simulink model "slexNLPClassificationLinearPredictExample"  (R2023a)
settings: Solver=FixedStepDiscrete  StartTime=0.0  StopTime=nlp.time(end)  FixedStep=1  RelTol=1e-3
PreLoadFcn:
  | if ~exist("linearMdl","var")
  | 
  | load nlpdata
  | 
  | n = size(X,1);
  | rng("default") % For reproducibility
  | shflidx = randperm(n);
  | X = X(shflidx,:);
  | Y = Y(shflidx);
  | 
  | Ystats = Y == "stats";
  | c = cvpartition(Ystats,Holdout=0.1);
  | idxPrsnt = training(c);
  | idxFtr = test(c);
  | 
  | prsntX = X(idxPrsnt,:);
  | prsntY = Ystats(idxPrsnt);
  | ftrX = X(idxFtr,:);
  | ftrY = Ystats(idxFtr);
  | 
  | linearMdl = fitclinear(prsntX,prsntY);
  | 
  | [nftrX,p] = size(ftrX);
  | nlp.time = (1:nftrX)' - 1;
  | nlp.signals(1).values = full(ftrX);
  | nlp.signals(1).dimensions = p;
  | 
  | end
libraries: statsLibrary x1
settings Model: Creator=The MathWorks, Inc.  LastModifiedBy=The MathWorks, Inc.
settings DataIOCC: ExternalInput=nlp  LoadExternalInput=on
settings OptimizationCC: ReuseModelBlockBuffer=off

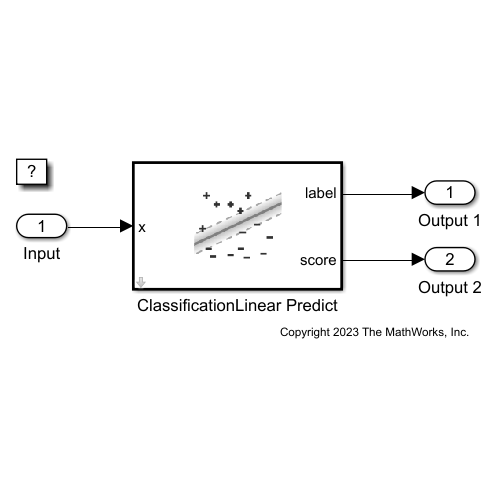
[thumbnail: Simulink's stored preview of the top-level diagram]
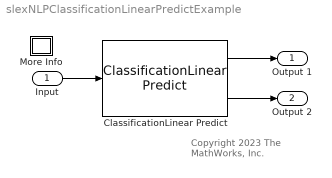
== system slexNLPClassificationLinearPredictExample ==
  note: Copyright 2023 The MathWorks, Inc.
  Input : Inport
  ClassificationLinear Predict : statsLibrary/Classification/ClassificationLinear Predict  TrainedLearner=linearMdl  ShowOutputScore=on  LabelDataTypeStr=Inherit: Inherit via back propagation  LabelOutMin=[]  LabelOutMax=[]  ScoreOutMin=[]  ScoreOutMax=[]  RawScoreOutMin=[]  RawScoreOutMax=[]  InnerProductOutMin=[]  InnerProductOutMax=[]  LinearSumOutMin=[]  LinearSumOutMax=[]  StoredEnumName=linearMdl_enumLabels
      settings: LibrarySourceBlock=statsLibrary/Classification/ClassificationSVM Predict1
  More Info : Subsystem
      settings: OpenFcn=showExample('stats/PredictClassLabelsUsingClassificationLinearPredictBlockExample')
      mask Display: disp('?')
  Output 1 : Outport
  Output 2 : Outport  Port=2
  wires:
  Input/1 -> ClassificationLinear Predict/1
  ClassificationLinear Predict/1 -> Output 1/1
  ClassificationLinear Predict/2 -> Output 2/1

== system slexNLPClassificationLinearPredictExample/More Info ==
